simulink model "DCMotorGenset"  (R2021a)
settings: Solver=VariableStepAuto  StartTime=0.0  StopTime=tEnd  RelTol=1e-3
values from neighbouring files (symbols this model uses):
  b = .002    (= 0.002)    [main.m]
  etaGenGR = 0.93    [main.m]
  GRgen = 1.4    [main.m]
  initialGasVolume = 5    [main.m]
  Jm = 5    [main.m]
  k_gal2kWh = 32.3    [main.m]
  k_hr2s = 3600    [main.m]
  k_kW2W = 1000    [main.m]
  k_m32gal = 264.172    [main.m]
  k_rpm2rps = 2*pi()/60    [main.m]
  k_rps2rpm = 60/(2*pi)    (= 9.54929658551)    [main.m]
  k_W2kW = 1/1000    (= 0.001)    [main.m]
  KD_DC = 0.02    [main.m]
  ke = kt    (= 3)    [main.m]
  KI_DC = 0.1    [main.m]
  KP_DC = 5    [main.m]
  kt = 3    [main.m]
  La = .01    (= 0.01)    [main.m]
  motorSpeedCommand = 800    [main.m]
  Ra = .06    (= 0.06)    [main.m]
  torqueCommand = 65    [main.m]
libraries: autolibsharedmappedengines x1, simulink x1
(part 3 of 3)

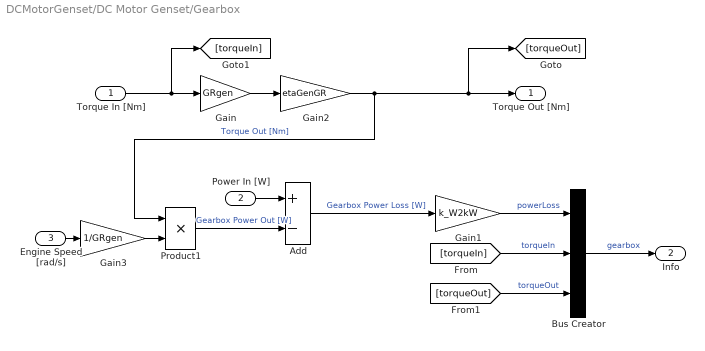
== system DCMotorGenset/DC Motor Genset/Gearbox ==
  Torque In [Nm] : Inport
  Power In [W] : Inport  Port=2
  Engine Speed [rad/s] : Inport  Port=3
  Add : Sum  Inputs=+-
  Bus Creator : BusCreator  Inputs=3
  Gain : Gain  Gain=GRgen
  Gain1 : Gain  Gain=k_W2kW
  Gain2 : Gain  Gain=etaGenGR
  Gain3 : Gain  Gain=1/GRgen
  Product1 : Product
  Torque Out [Nm] : Outport
  Info : Outport  Port=2
  wires:
  Gain3/1 -> Product1/2
  Bus Creator/1 -> Info/1  "gearbox"
  [torqueOut] -> Bus Creator/3  "torqueOut"
  [torqueIn] -> Bus Creator/2  "torqueIn"
  Gain1/1 -> Bus Creator/1  "powerLoss"
  Torque In [Nm]/1 -> Gain/1, [torqueIn]
  Add/1 -> Gain1/1  "Gearbox Power Loss [W]"
  Power In [W]/1 -> Add/1
  Gain/1 -> Gain2/1
  Engine Speed [rad/s]/1 -> Gain3/1
  Product1/1 -> Add/2  "Gearbox Power Out [W]"
  Gain2/1 -> Product1/1, Torque Out [Nm]/1, [torqueOut]  "Torque Out [Nm]"

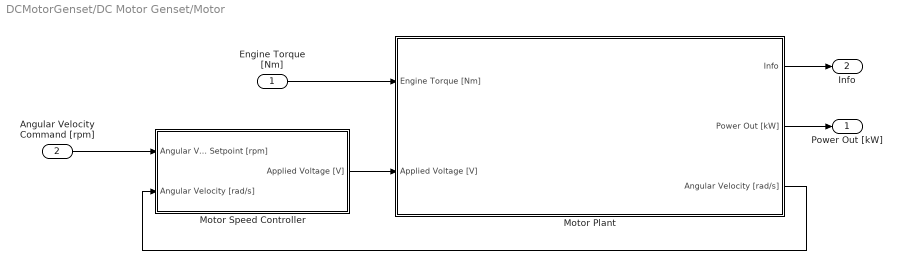
== system DCMotorGenset/DC Motor Genset/Motor ==
  Engine Torque [Nm] : Inport
  Angular Velocity Command [rpm] : Inport  Port=2
  Motor Plant : Subsystem
  Motor Speed Controller : Subsystem
  Power Out [kW] : Outport
  Info : Outport  Port=2
  wires:
  Engine Torque [Nm]/1 -> Motor Plant/1(Engine Torque [Nm])
  Motor Plant/2(Power Out [kW]) -> Power Out [kW]/1
  Motor Plant/1(Info) -> Info/1
  Motor Plant/3(Angular Velocity [rad/s]) -> Motor Speed Controller/2(Angular Velocity [rad/s])
  Motor Speed Controller/1(Applied Voltage [V]) -> Motor Plant/2(Applied Voltage [V])
  Angular Velocity Command [rpm]/1 -> Motor Speed Controller/1(Angular Velocity Setpoint [rpm])

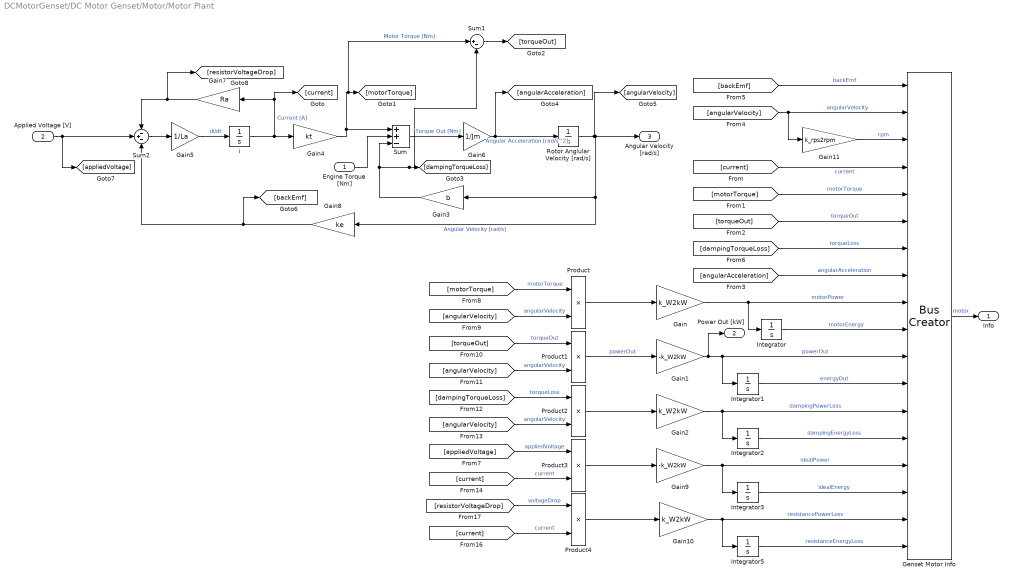
== system DCMotorGenset/DC Motor Genset/Motor/Motor Plant ==
  Engine Torque [Nm] : Inport
  Applied Voltage [V] : Inport  Port=2
  Gain : Gain  Gain=k_W2kW
  Gain1 : Gain  Gain=-k_W2kW
  Gain10 : Gain  Gain=k_W2kW
  Gain11 : Gain  Gain=k_rps2rpm
  Gain2 : Gain  Gain=k_W2kW
  Gain3 : Gain  Gain=b
  Gain4 : Gain  Gain=kt
  Gain5 : Gain  Gain=1/La
  Gain6 : Gain  Gain=1/Jm
  Gain7 : Gain  Gain=Ra
  Gain8 : Gain  Gain=ke
  Gain9 : Gain  Gain=-k_W2kW
  Genset Motor Info : BusCreator  Inputs=18
  Integrator{,1..3,5} (5 alike) : Integrator
  Product{,1..4} (5 alike) : Product
  Rotor Anglular Velocity [rad/s] : Integrator
  Sum : Sum  Inputs=++-
  Sum1 : Sum  Inputs=|+-
  Sum2 : Sum  Inputs=-+-
  i : Integrator
  Info : Outport
  Power Out [kW] : Outport  Port=2
  Angular Velocity [rad/s] : Outport  Port=3
  wires:
  Sum1/1 -> [torqueOut]
  Engine Torque [Nm]/1 -> Sum/2
  [angularVelocity] -> Product/2  "angularVelocity"
  [angularVelocity] -> Genset Motor Info/2, Gain11/1  "angularVelocity"
  [motorTorque] -> Product/1  "motorTorque"
  [current] -> Product4/2  "current"
  Gain1/1 -> Power Out [kW]/1, Integrator1/1, Genset Motor Info/11  "powerOut"
  Integrator/1 -> Genset Motor Info/10  "motorEnergy"
  Gain2/1 -> Genset Motor Info/13, Integrator2/1  "dampingPowerLoss"
  Product4/1 -> Gain10/1
  Gain9/1 -> Integrator3/1, Genset Motor Info/15  "idealPower"
  [dampingTorqueLoss] -> Product2/1  "torqueLoss"
  [resistorVoltageDrop] -> Product4/1  "voltageDrop"
  Gain11/1 -> Genset Motor Info/3  "rpm"
  [motorTorque] -> Genset Motor Info/5  "motorTorque"
  [backEmf] -> Genset Motor Info/1  "backEmf"
  [current] -> Product3/2  "current"
  Product1/1 -> Gain1/1  "powerOut"
  Product/1 -> Gain/1
  [current] -> Genset Motor Info/4  "current"
  [angularVelocity] -> Product1/2  "angularVelocity"
  Product3/1 -> Gain9/1
  Integrator1/1 -> Genset Motor Info/12  "energyOut"
  Gain/1 -> Genset Motor Info/9, Integrator/1  "motorPower"
  [angularAcceleration] -> Genset Motor Info/8  "angularAcceleration"
  Product2/1 -> Gain2/1
  Integrator5/1 -> Genset Motor Info/18  "resistanceEnergyLoss"
  [angularVelocity] -> Product2/2  "angularVelocity"
  [appliedVoltage] -> Product3/1  "appliedVoltage"
  [torqueOut] -> Product1/1  "torqueOut"
  [dampingTorqueLoss] -> Genset Motor Info/7  "torqueLoss"
  [torqueOut] -> Genset Motor Info/6  "torqueOut"
  Integrator3/1 -> Genset Motor Info/16  "idealEnergy"
  Gain10/1 -> Integrator5/1, Genset Motor Info/17  "resistancePowerLoss"
  Integrator2/1 -> Genset Motor Info/14  "dampingEnergyLoss"
  Genset Motor Info/1 -> Info/1  "motor"
  Gain7/1 -> Sum2/1, [resistorVoltageDrop]
  Gain8/1 -> Sum2/3, [backEmf]
  Applied Voltage [V]/1 -> [appliedVoltage], Sum2/2
  Sum2/1 -> Gain5/1
  Rotor Anglular Velocity [rad/s]/1 -> [angularVelocity], Gain3/1, Gain8/1, Angular Velocity [rad/s]/1  "Angular Velocity [rad/s]"
  Gain5/1 -> i/1  "di/dt"
  Gain3/1 -> [dampingTorqueLoss], Sum1/2, Sum/3
  i/1 -> Gain7/1, [current], Gain4/1  "Current [A]"
  Gain6/1 -> [angularAcceleration], Rotor Anglular Velocity [rad/s]/1  "Angular Acceleration [rad/s^2]"
  Gain4/1 -> Sum/1, [motorTorque], Sum1/1  "Motor Torque [Nm]"
  Sum/1 -> Gain6/1  "Torque Out [Nm]"

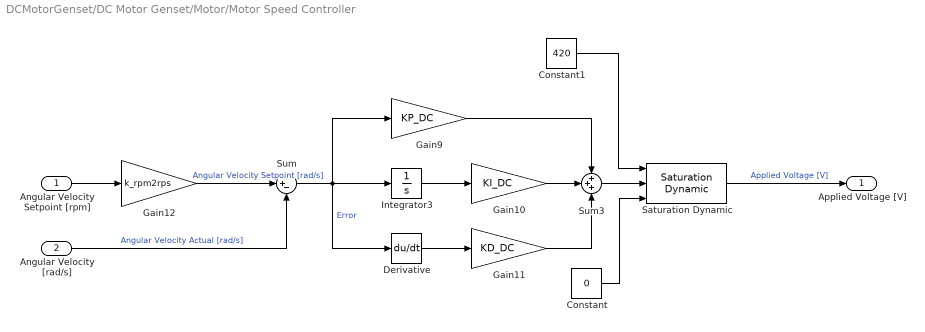
== system DCMotorGenset/DC Motor Genset/Motor/Motor Speed Controller ==
  Angular Velocity Setpoint [rpm] : Inport
  Angular Velocity [rad/s] : Inport  Port=2
  Constant : Constant  Value=0
  Constant1 : Constant  Value=420
  Derivative : Derivative
  Gain10 : Gain  Gain=KI_DC
  Gain11 : Gain  Gain=KD_DC
  Gain12 : Gain  Gain=k_rpm2rps
  Gain9 : Gain  Gain=KP_DC
  Integrator3 : Integrator
  Saturation Dynamic : simulink/Discontinuities/Saturation Dynamic  OutMin=[]  OutMax=[]  OutDataTypeStr=Inherit: Same as second input  OutDataType=fixdt(1, 16)  OutScaling=2^-10  DoSatur=off
  Sum : Sum  Inputs=|+-
  Sum3 : Sum  Inputs=+++
  Applied Voltage [V] : Outport
  wires:
  Sum3/1 -> Saturation Dynamic/2
  Constant/1 -> Saturation Dynamic/3
  Constant1/1 -> Saturation Dynamic/1
  Saturation Dynamic/1 -> Applied Voltage [V]/1  "Applied Voltage [V]"
  Angular Velocity [rad/s]/1 -> Sum/2  "Angular Velocity Actual [rad/s]"
  Gain12/1 -> Sum/1  "Angular Velocity Setpoint [rad/s]"
  Gain9/1 -> Sum3/1
  Gain11/1 -> Sum3/3
  Sum/1 -> Derivative/1, Integrator3/1, Gain9/1  "Error"
  Gain10/1 -> Sum3/2
  Angular Velocity Setpoint [rpm]/1 -> Gain12/1
  Integrator3/1 -> Gain10/1
  Derivative/1 -> Gain11/1
